simulink model "Task4_DoorSignal"  (R2025a)
settings: Solver=ode4  StartTime=0.0  StopTime=10.0  FixedStep=1e-5  RelTol=1e-3
model workspace (MAT data in the model file):
  h = Simulink.Parameter
  h.Value = 0.03
  h.Complexity = 'real'
  h.Dimensions = [1 1]
  h.DataType = 'auto'
  l = Simulink.Parameter
  l.Value = 0.05
  l.Complexity = 'real'
  l.Dimensions = [1 1]
  l.DataType = 'auto'
  v = Simulink.Parameter
  v.Value = 1
  v.Complexity = 'real'
  v.Dimensions = [1 1]
  v.DataType = 'auto'
libraries: simulink x3
settings Model: Creator=randi  LastModifiedBy=randi

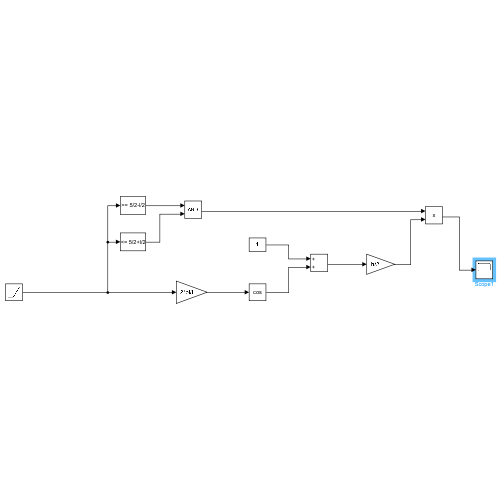
[thumbnail: Simulink's stored preview of the top-level diagram]
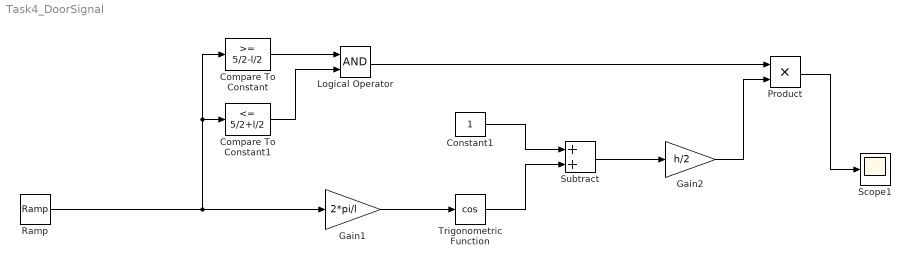
== system Task4_DoorSignal ==
  Compare To Constant : simulink/Logic and Bit Operations/Compare To Constant  relop=>=  const=5/2-l/2  OutDataTypeStr=boolean
  Compare To Constant1 : simulink/Logic and Bit Operations/Compare To Constant  relop=<=  const=5/2+l/2  OutDataTypeStr=boolean
  Constant1 : Constant
  Gain1 : Gain  Gain=2*pi/l
  Gain2 : Gain  Gain=h/2
  Logical Operator : Logic  AllPortsSameDT=off  OutDataTypeStr=boolean
  Product : Product
  Ramp : simulink/Sources/Ramp  slope=v  start=0  InitialOutput=0
  Scope1 : Scope
      settings: ActiveDisplayYMinimum=-0.00034063545103461476  ActiveDisplayYMaximum=0.030335849008314396
  Subtract : Sum
  Trigonometric Function : Trigonometry  Operator=cos
  wires:
  Subtract/1 -> Gain2/1
  Trigonometric Function/1 -> Subtract/2
  Constant1/1 -> Subtract/1
  Compare To Constant/1 -> Logical Operator/1
  Compare To Constant1/1 -> Logical Operator/2
  Logical Operator/1 -> Product/1
  Ramp/1 -> Compare To Constant/1, Compare To Constant1/1, Gain1/1
  Gain2/1 -> Product/2
  Product/1 -> Scope1/1
  Gain1/1 -> Trigonometric Function/1
